simulink model "GFo_29bus"  (R2017b)
settings: Solver=ode1  StartTime=0.0  StopTime=4.5  FixedStep=Time_Step  RelTol=1e-3  EnableMultiTasking=on
PreLoadFcn:
  | Init_29bus;
InitFcn:
  | Init_29bus;
undefined symbols (not defined in the file): C_line, D1, D11, Delta, DX_DR, fb, fn, I_thresh_pu, Kp_Rvi_pu, Time_Step, VSC01_Cf, VSC01_Cf_pu, VSC01_Delta_P_Time_Step, VSC01_Delta_P_Value, VSC01_id0, VSC01_Lf, VSC01_Lf_pu, VSC01_Lt_pu, VSC01_mp1, VSC01_mp2, VSC01_mp3, VSC01_Pn, VSC01_R, VSC01_Rf, VSC01_Rf_pu, VSC01_Rt_pu, VSC01_Rv, VSC01_Sn, VSC01_T1, VSC01_T2, VSC01_Tr_PLL, VSC01_Udc_n, VSC01_Udcb, VSC01_Un1, VSC01_Un2, VSC01_W_LF, VSC01_wc1, VSC01_wc2, VSC01_wc3
libraries: powerlib x183, sps_avr x6, simulink x4, powerlib_meascontrol x2
(part 1 of 7)
Description:
  | Copyright 2008-2017 The MathWorks, Inc.
settings Model: Creator=MathWorks  LastModifiedBy=Frederic_Colas
settings DataIOCC: SaveFormat=StructureWithTime  SignalLoggingSaveFormat=ModelDataLogs  SaveOutput=off  SignalLogging=off  DSMLogging=off  SaveTime=off
settings OptimizationCC: ExpressionDepthLimit=2147483647  LifeSpan=inf
settings DebuggingCC: UnderspecifiedInitializationDetection=Classic  MergeDetectMultiDrivingBlocksExec=none  SolverPrmCheckMsg=warning  FcnCallInpInsideContextMsg=warning  UnconnectedInputMsg=none  UnconnectedOutputMsg=none  UnconnectedLineMsg=none  StateNameClashWarn=warning  SFUnexpectedBacktrackingDiag=warning  SFNoUnconditionalDefaultTransitionDiag=warning  SFExecutionAtInitializationDiag=none
settings HardwareCC: ProdBitPerPointer=32  ProdBitPerSizeT=32  ProdBitPerPtrDiffT=32  ProdLargestAtomicFloat=None  ProdIntDivRoundTo=Undefined  ProdEndianess=Unspecified  ProdWordSize=32  ProdHWDeviceType=32-bit Generic
settings ModelReferenceCC: PropagateSignalLabelsOutOfModel=off
settings CodeAppCC: StateflowObjectComments=on
settings GRTTargetCC: TargetLangStandard=C89/C90 (ANSI)  GeneratePreprocessorConditionals=Disable all  CombineOutputUpdateFcns=off  GRTInterface=on
settings ConfigComp: CovMetricSettings=dw  CovHtmlReporting=on  CovSaveCumulativeToWorkspaceVar=on  CovSaveSingleToWorkspaceVar=on  CovExternalEMLEnable=off  CovSFcnEnable=off
settings SimscapeCC: SimscapeNormalizeSystem=off

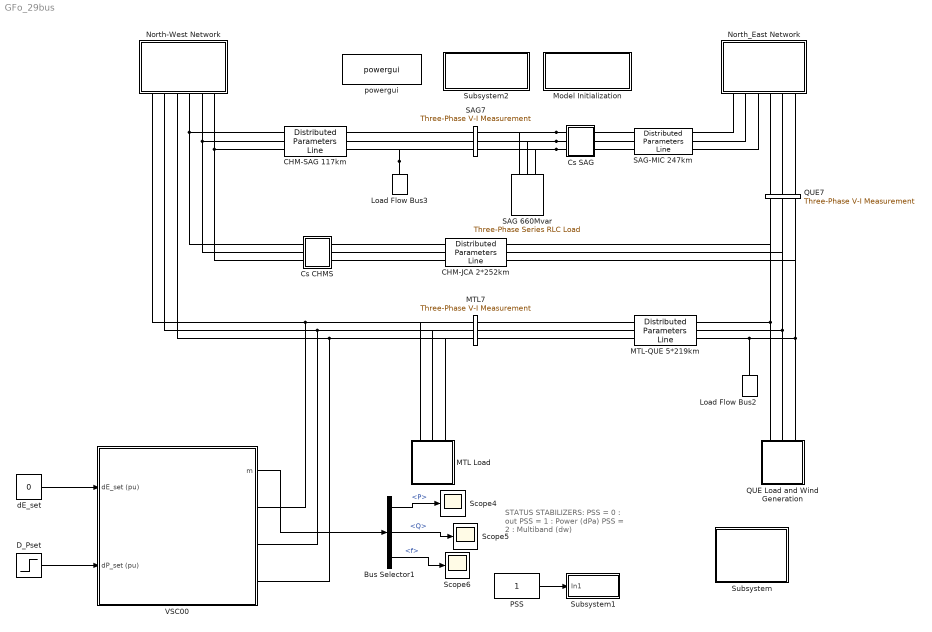
== system GFo_29bus ==
  note: STATUS STABILIZERS:
      | PSS = 0 :  out
      | PSS = 1 :  Power (dPa)
      | PSS = 2 :  Multiband (dw)
  Bus Selector1 : BusSelector  OutputSignals=control.P,control.Q,control.f
  CHM-JCA 2*252km : powerlib/Elements/Distributed Parameters Line  Phases=3  Frequency=60  Resistance="[0.01273  0.3864]/2"  Inductance="[0.9337e-3  4.1264e-3]/2"  Capacitance=[12.74e-9 7.751e-9]*2  Length=252  x1=[-0.00144 -3.02391793740978e-08 0 0;-0.0014 -3.09921305238755e-08 0 0;-0.00136 -3.17380343304367e-08 0 0;-0.00132 -3.24767211816884e-08 0 0;-0.00128 -3.32080231066107e-08 0 0;-0.00124 -3.39317738134523e-08 0 0;-0.0012 -3.46478087275439e-08 0 0;-0.00116 -3.53559650287208e-08 0 0;-0.00112 -3.60560816883471e-08 0 0;-0.00108 -3.67479995059318e-08 0 0;-0.00104 -3.74315611453301e-08 0 0;-0.001 -3.810661117052e-08 0 0;-0.00096 -3.87729960809472e-08 0 0;-0.00092 -3.94305643464296e-08 0 0;-0.00088 -4.00791664416144e-08 265077.167906972 -634102.982105748;-0.00084 -4.07186548799783e-08 274608.708093749 -630033.76126445;-0.0008 -4.13488842473653e-08 284077.80462843 -625821.276179022;-0.00076 -4.1969711235052e-08 293482.30432012 -621466.484732242;-0.00072 -4.25809946723352e-08 302820.068666693 -616970.377166134;-0.00068 -4.31825955586328e-08 312088.974341059 -612333.975856784;-0.00064 -4.37743770950913e-08 321286.913674001 -607558.335081867;-0.0006 -4.43562047156924e-08 330411.795133434 -602644.540780912;-0.00056 -4.49279461178528e-08 339461.543800003 -597593.710308369;-0.00052 -4.54894712925081e-08 348434.101838904 -592406.992179531;-0.00048 -4.6040652553676e-08 357327.428967815 -587085.565809372;-0.00044 -4.65813645674909e-08 366139.502920839 -581630.641244357;-0.0004 -4.71114843807037e-08 374868.319908351 -576043.458887293;-0.00036 -4.76308914486404e-08 383511.895072643 -570325.289215265;-0.00032 -4.81394676626131e-08 392068.262939261 -564477.432490745;-0.00028 -4.86370973767763e-08 400535.477863939 -558501.218465923;-0.00024 -4.91236674344246e-08 408911.614475022 -552398.006080331;-0.0002 -4.95990671937227e-08 417194.768111276 -546169.183151834;-0.00016 -5.00631885528651e-08 425383.055254997 -539816.166061051;-0.00012 -5.05159259746572e-08 433474.6139603 -533340.399429281;-8e-05 -5.09571765105133e-08 441467.604276514 -526743.355790014;-4e-05 -5.1386839823867e-08 449360.208666571 -520026.53525408]  x2=[-0.00144 -2.32746545563594e-08 0 0;-0.0014 -2.37082501505167e-08 0 0;-0.00136 -2.41364546930411e-08 0 0;-0.00132 -2.45591708139122e-08 0 0;-0.00128 -2.49763023911295e-08 0 0;-0.00124 -2.53877545725695e-08 0 0;-0.0012 -2.57934337975543e-08 0 0;-0.00116 -2.61932478181267e-08 0 0;-0.00112 -2.65871057200262e-08 0 0;-0.00108 -2.69749179433624e-08 0 0;-0.00104 -2.73565963029801e-08 0 0;-0.001 -2.77320540085117e-08 0 0;-0.00096 -2.81012056841128e-08 0 0;-0.00092 -2.84639673878759e-08 0 0;-0.00088 -2.88202566309177e-08 37345.2323788199 -657445.860812689;-0.00084 -2.9169992396137e-08 47254.6604347232 -656807.985703751;-0.0008 -2.95130951566367e-08 57153.3431883505 -656020.758122934;-0.00076 -2.98494868938078e-08 67039.0297646062 -655084.357079001;-0.00072 -3.01790911150703e-08 76909.4722436134 -653998.995501477;-0.00068 -3.05018328712667e-08 86762.4261718714 -652764.920192222;-0.00064 -3.08176387737047e-08 96595.6510726253 -651382.41176932;-0.0006 -3.11264370108456e-08 106406.910955331 -649851.784603265;-0.00056 -3.14281573646332e-08 116193.974824099 -648173.386745474;-0.00052 -3.17227312264609e-08 125954.617185006 -646347.599849146;-0.00048 -3.2010091612773e-08 135686.618552152 -644374.839082477;-0.00044 -3.22901731802955e-08 145387.765952351 -642255.553034253;-0.0004 -3.25629122408955e-08 155055.853428343 -639990.223611844;-0.00036 -3.28282467760625e-08 164688.68254041 -637579.365931627;-0.00032 -3.30861164510113e-08 174284.062866282 -635023.528201848;-0.00028 -3.33364626284017e-08 183839.81249922 -632323.291597964;-0.00024 -3.35792283816718e-08 193353.758544162 -629479.270130496;-0.0002 -3.38143585079829e-08 202823.737611824 -626492.110505397;-0.00016 -3.40417995407718e-08 212247.59631063 -623362.491977008;-0.00012 -3.42614997619092e-08 221623.19173638 -620091.126193592;-8e-05 -3.44734092134592e-08 230948.391959526 -616678.757035518;-4e-05 -3.46774797090402e-08 240221.076509955 -613126.160446105]  x3=[-0.00144 -1.32107929850916e-10 0 0;-0.0014 -1.33450786607546e-10 0 0;-0.00136 -1.34763297806132e-10 0 0;-0.00132 -1.36045164992946e-10 0 0;-0.00128 -1.37296096682445e-10 0 0;-0.00124 -1.38515808423548e-10 0 0;-0.0012 -1.39704022864326e-10 0 0;-0.00116 -1.4086046981506e-10 0 0;-0.00112 -1.41984886309688e-10 0 0;-0.00108 -1.43077016665594e-10 0 0;-0.00104 -1.44136612541754e-10 0 0;-0.001 -1.45163432995204e-10 0 0;-0.00096 -1.46157244535826e-10 0 0;-0.00092 -1.47117821179447e-10 0 0;-0.00088 -1.48044944499222e-10 455.51432786146 206.852095953411;-0.00084 -1.48938403675303e-10 452.343644908568 213.697505315651;-0.0008 -1.49797995542779e-10 449.07010291167 220.494321708032;-0.00076 -1.50623524637871e-10 445.694446245985 227.240999593118;-0.00072 -1.51414803242382e-10 442.217442506729 233.936004834539;-0.00068 -1.52171651426382e-10 438.639882334567 240.57781504584;-0.00064 -1.5289389708912e-10 434.962579235833 247.164919936653;-0.0006 -1.5358137599816e-10 431.186369397537 253.695821656133;-0.00056 -1.54233931826728e-10 427.312111497233 260.169035133548;-0.00052 -1.54851416189255e-10 423.340686507758 266.583088415975;-0.00048 -1.55433688675123e-10 419.272997496905 272.936523003011;-0.00044 -1.55980616880589e-10 415.109969422078 279.227894178421;-0.0004 -1.56492076438896e-10 410.85254891996 285.455771338653;-0.00036 -1.5696795104855e-10 406.501704091259 291.618738318149;-0.00032 -1.57408132499771e-10 402.05842428057 297.715393711364;-0.00028 -1.5781252069909e-10 397.523719851403 303.744351191437;-0.00024 -1.5818102369212e-10 392.89862195644 309.704239825429;-0.0002 -1.58513557684458e-10 388.184182303058 315.593704386061;-0.00016 -1.58810047060741e-10 383.381472914178 321.411405659879;-0.00012 -1.59070424401841e-10 378.491585884498 327.156020751784;-8e-05 -1.59294630500198e-10 373.515633132161 332.826243385843;-4e-05 -1.59482614373277e-10 368.454746145911 338.420784202328]  x4=[-0.00144 5.44626892198022e-11 0 0;-0.0014 5.22863667553336e-11 0 0;-0.00136 5.00981548219633e-11 0 0;-0.00132 4.78985510002146e-11 0 0;-0.00128 4.56880554610279e-11 0 0;-0.00124 4.34671708520264e-11 0 0;-0.0012 4.12364021832181e-11 0 0;-0.00116 3.89962567121609e-11 0 0;-0.00112 3.67472438286167e-11 0 0;-0.00108 3.44898749387207e-11 0 0;-0.00104 3.22246633486916e-11 0 0;-0.001 2.99521241481107e-11 0 0;-0.00096 2.76727740927946e-11 0 0;-0.00092 2.53871314872896e-11 0 0;-0.00088 2.30957160670137e-11 190.753638286441 -10030.4733717918;-0.00084 2.07990488800732e-11 341.981891608961 -10026.4567433659;-0.0008 1.84976521687807e-11 493.132381198454 -10020.1601851409;-0.00076 1.6192049250902e-11 644.170736737055 -10011.5851289001;-0.00072 1.38827644006579e-11 795.062613405215 -10000.7335245372;-0.00068 1.15703227295089e-11 945.773699691414 -9987.60783961345;-0.00064 9.2552500667495e-12 1096.26972519431 -9972.21105879643;-0.0006 6.93807283993878e-12 1246.51646841552 -9954.54668318134;-0.00056 4.61931795519565e-12 1396.47976454132 -9934.61872949484;-0.00052 2.29951267738481e-12 1546.12551321138 -9912.43172918176;-0.00048 -2.08154897787282e-14 1695.41968627296 -9887.99072737463;-0.00044 -2.34113892367939e-12 1844.32833551856 -9861.3012817465;-0.0004 -4.66093000277792e-12 1992.81760040548 -9832.36946124714;-0.00036 -6.97966122658797e-12 2140.85371575538 -9801.20184472303;-0.00032 -9.29680533562514e-12 2288.40301943227 -9767.8055194214;-0.00028 -1.16118354313012e-11 2435.43195999687 -9732.18807937862;-0.00024 -1.39242250957364e-11 2581.90710433605 -9694.35762369341;-0.0002 -1.62334485114622e-11 2727.79514526512 -9654.32275468515;-0.00016 -1.85389805809879e-11 2873.06290910166 -9612.0925759378;-0.00012 -2.08402970462027e-11 3017.67736320891 -9567.67669022985;-8e-05 -2.31368746075884e-11 3161.60562350711 -9521.08519735066;-4e-05 -2.54281910432121e-11 3304.81496195104 -9472.32869180394]  x5=0.00142516474882927  V1=ones(3,3)  V2=ones(3,3)  I1=ones(3,3)  I2=ones(3,3)  nHarmo=1  Measurements=None
      settings: AttributesFormatString=\n  SourceProductName=Simscape Power Systems
  CHM-SAG 117km : powerlib/Elements/Distributed Parameters Line  Phases=3  Frequency=60  Resistance="[0.01273  0.3864]"  Inductance="[0.9337e-3  4.1264e-3]"  Capacitance=[12.74e-9 7.751e-9]  Length=117  x1=[-0.00068 -4.23803703751889e-08 0 0;-0.00064 -4.29595449086164e-08 0 0;-0.0006 -4.35289508119991e-08 0 0;-0.00056 -4.40884586073449e-08 0 0;-0.00052 -4.4637941067406e-08 0 0;-0.00048 -4.51772732446096e-08 0 0;-0.00044 -4.57063324994695e-08 290815.275178508 -619240.212617567;-0.0004 -4.62249985284737e-08 300119.775081889 -614784.578978232;-0.00036 -4.673315339144e-08 309356.030336538 -610189.148627313;-0.00032 -4.72306815383346e-08 318521.940697662 -605454.966526043;-0.00028 -4.77174698355474e-08 327615.421916287 -600583.109186607;-0.00024 -4.81934075916175e-08 336634.406213204 -595574.68442735;-0.0002 -4.86583865824036e-08 345576.842749159 -590430.831120871;-0.00016 -4.91123010756929e-08 354440.698091201 -585152.718935054;-0.00012 -4.9555047855244e-08 363223.956675063 -579741.548067093;-8e-05 -4.99865262442574e-08 371924.621263487 -574198.54897058;-4e-05 -5.04066381282682e-08 380540.713400378 -568524.982075709]  x2=[-0.00068 -2.9225958888399e-08 0 0;-0.00064 -2.96330480824069e-08 0 0;-0.0006 -3.00333989768254e-08 0 0;-0.00056 -3.04269205353136e-08 0 0;-0.00052 -3.08135232744627e-08 0 0;-0.00048 -3.11931192841436e-08 0 0;-0.00044 -3.15656222474974e-08 342715.137788314 -587516.495420752;-0.0004 -3.19309474605624e-08 351535.375086538 -582281.875650636;-0.00036 -3.22890118515356e-08 360275.676271978 -576914.850003381;-0.00032 -3.26397339996624e-08 368934.05387552 -571416.638894338;-0.00028 -3.29830341537507e-08 377508.539056762 -565788.492569297;-0.00024 -3.3318834250306e-08 385997.182051718 -560031.690820198;-0.0002 -3.36470579312822e-08 394398.052616172 -554147.542694114;-0.00016 -3.39676305614447e-08 402709.240464606 -548137.386195587;-0.00012 -3.42804792453419e-08 410928.855704575 -542002.587982374;-8e-05 -3.45855328438809e-08 419055.029266456 -535744.543054685;-4e-05 -3.48827219905042e-08 427085.913328459 -529364.67443797]  x3=[-0.00068 -9.13993390137404e-11 0 0;-0.00064 -9.10085517468096e-11 0 0;-0.0006 -9.0597069920036e-11 0 0;-0.00056 -9.01649871008385e-11 0 0;-0.00052 -8.97124015411239e-11 0 0;-0.00048 -8.92394161549457e-11 0 0;-0.00044 -8.87461384951018e-11 1711.45288043998 -3591.83174853406;-0.0004 -8.82326807286782e-11 1765.41999013625 -3565.61618486843;-0.00036 -8.76991596115431e-11 1818.9856585511 -3538.58983083092;-0.00032 -8.71456964617978e-11 1872.13770531345 -3510.75883198137;-0.00028 -8.65724171321895e-11 1924.86404410625 -3482.12951684893;-0.00024 -8.5979451981494e-11 1977.15268541473 -3452.70839549296;-0.0002 -8.53669358448732e-11 2028.99173925279 -3422.50215802275;-0.00016 -8.47350080032144e-11 2080.36941786663 -3391.51767307621;-0.00012 -8.40838121514592e-11 2131.27403841518 -3359.761986258;-8e-05 -8.34134963659287e-11 2181.69402562672 -3327.24231853748;-4e-05 -8.27242130706519e-11 2231.61791443097 -3293.96606460664]  x4=[-0.00068 9.30343370038175e-12 0 0;-0.00064 7.45357527579132e-12 0 0;-0.0006 5.60202197246008e-12 0 0;-0.00056 3.74919481764209e-12 0 0;-0.00052 1.89551512825424e-12 0 0;-0.00048 4.14044150724481e-14 0 0;-0.00044 -1.81271571311628e-12 280.288551649878 -1025.23386773629;-0.0004 -3.66642364538403e-12 295.716038711893 -1020.89088180168;-0.00036 -5.51929786453271e-12 311.076282496852 -1016.31575408433;-0.00032 -7.3709170429434e-12 326.365790217779 -1011.50952492885;-0.00028 -9.22086013838259e-12 341.581085172469 -1006.47328723028;-0.00024 -1.10687064897436e-11 356.71870753406 -1001.20818618565;-0.0002 -1.29140359127014e-11 371.775215137769 -995.71541903353;-0.00016 -1.47564287952585e-11 386.747184263609 -989.996234781809;-0.00012 -1.65954661931615e-11 401.631210414913 -984.051933923662;-8e-05 -1.84307299251655e-11 416.423909092489 -977.883868141844;-4e-05 -2.02618026681243e-11 431.121916564223 -971.493440001321]  x5=0.000661683633385019  V1=ones(3,3)  V2=ones(3,3)  I1=ones(3,3)  I2=ones(3,3)  nHarmo=1  Measurements=None
      settings: AttributesFormatString=\n  SourceProductName=Simscape Power Systems
  Cs CHMS : Subsystem  mask{Xc=33/2}
      mask prompts: Xc "Condensator Reactance at  60Hz  (ohm):"
      mask help: Series Compensation
      mask init:
      | Cs=1/Xc/(2*pi*60);
      mask Display: disp('Cs')
  Cs SAG : Subsystem  mask{Xc=22}
      mask prompts: Xc "Condensator Reactance at  60Hz  (ohm):"
      mask help: Series Compensation
      mask init:
      | Cs=1/Xc/(2*pi*60);
      mask Display: disp('Cs')
  D_Pset : Step  Time=VSC01_Delta_P_Time_Step  After=VSC01_Delta_P_Value  SampleTime=0
  Load Flow Bus2 : powerlib/Measurements/Load Flow Bus  LConnTagsString=a  Phases=single  Connectors=on one side  ID=QUE7  Vbase=735e3  Vref=1  Vangle=0  VLF=1.016  VLFb=1  VLFc=1  angleLF=-12.43  angleLFb=0  angleLFc=0
      settings: AttributesFormatString=%<ID>\n%<Vbase>V\n%<VLF>pu\n%<angleLF>deg.  SourceProductName=Simscape Power Systems
  Load Flow Bus3 : powerlib/Measurements/Load Flow Bus  LConnTagsString=a  Phases=single  Connectors=on one side  ID=SAG7  Vbase=735e3  Vref=1  Vangle=0  VLF=1.034  VLFb=1  VLFc=1  angleLF=2.226  angleLFb=0  angleLFc=0
      settings: AttributesFormatString=%<ID>\n%<Vbase>V\n%<VLF>pu\n%<angleLF>deg.  SourceProductName=Simscape Power Systems
  MTL Load : Subsystem
  MTL-QUE 5*219km : powerlib/Elements/Distributed Parameters Line  Phases=3  Frequency=60  Resistance="[0.01273  0.3864]/5"  Inductance="[0.9337e-3  4.1264e-3]/5"  Capacitance=[12.74e-9 7.751e-9]*5  Length=219  x1=[-0.00124 -1.29467243971328e-07 -185501.595169669 -635267.89625739;-0.0012 -1.3225224728807e-07 -175901.255117953 -637992.862327818;-0.00116 -1.35007177584273e-07 -166260.91663773 -640572.754323168;-0.00112 -1.37731408412545e-07 -156582.771858837 -643006.985598249;-0.00108 -1.4042432030629e-07 -146869.021507936 -645295.002629861;-0.00104 -1.43085300920565e-07 -137121.874408088 -647436.285142663;-0.001 -1.45713745171325e-07 -127343.546976489 -649430.346227476;-0.00096 -1.48309055373016e-07 -117536.262720471 -651276.732452005;-0.00092 -1.50870641374477e-07 -107702.2517319 -652975.023963946;-0.00088 -1.53397920693143e-07 -97843.7501800699 -654524.834586454;-0.00084 -1.55890318647491e-07 -87962.9998032174 -655925.81190596;-0.0008 -1.58347268487719e-07 -78062.2473987702 -657177.637352301;-0.00076 -1.60768211524621e-07 -68143.7443124447 -658280.026271167;-0.00072 -1.63152597256629e-07 -58209.7459263092 -659232.727988824;-0.00068 -1.65499883494989e-07 -48262.5111459295 -660035.525869117;-0.00064 -1.67809536487052e-07 -38304.3018867134 -660688.237362731;-0.0006 -1.70081031037646e-07 -28337.3825595705 -661190.714048703;-0.00056 -1.72313850628499e-07 -18364.0195560047 -661542.841668165;-0.00052 -1.74507487535689e-07 -8386.48073275649 -661744.540150334;-0.00048 -1.76661442945103e-07 1592.96510388849 -661795.763630715;-0.00044 -1.78775227065854e-07 11572.048714006 -661696.50046153;-0.0004 -1.80848359241663e-07 21548.500940039 -661446.773214367;-0.00036 -1.82880368060149e-07 31520.0532227846 -661046.63867505;-0.00032 -1.84870791460032e-07 41484.4381172447 -660496.187830721;-0.00028 -1.86819176836195e-07 51439.3898082235 -659795.545849157;-0.00024 -1.88725081142605e-07 61382.6446255543 -658944.8720503;-0.0002 -1.90588070993059e-07 71311.9415588386 -657944.359870038;-0.00016 -1.92407722759731e-07 81225.0227715805 -656794.236816212;-0.00012 -1.94183622669501e-07 91119.6341145989 -655494.764416886;-8e-05 -1.95915366898044e-07 100993.525638602 -654046.238160878;-4e-05 -1.97602561661656e-07 110844.452105806 -652448.987430567]  x2=[-0.00124 -2.53877545725695e-08 -51950.9609807774 -656453.169013363;-0.0012 -2.57934337975543e-08 -42046.3485068077 -657161.91059321;-0.00116 -2.61932478181267e-08 -32132.1750557799 -657721.219221712;-0.00112 -2.65871057200262e-08 -22210.6950252404 -658130.967716908;-0.00108 -2.69749179433624e-08 -12284.1644741892 -658391.062905526;-0.00104 -2.73565963029801e-08 -2354.84061007062 -658501.445644162;-0.001 -2.77320540085117e-08 7575.01872449539 -658462.090832732;-0.00096 -2.81012056841128e-08 17503.1555651277 -658273.007420183;-0.00092 -2.84639673878759e-08 27427.3123391252 -657934.238402451;-0.00088 -2.88202566309177e-08 37345.2323788199 -657445.860812689;-0.00084 -2.9169992396137e-08 47254.6604347232 -656807.985703751;-0.0008 -2.95130951566367e-08 57153.3431883505 -656020.758122934;-0.00076 -2.98494868938078e-08 67039.0297646062 -655084.357079001;-0.00072 -3.01790911150703e-08 76909.4722436134 -653998.995501477;-0.00068 -3.05018328712667e-08 86762.4261718714 -652764.920192222;-0.00064 -3.08176387737047e-08 96595.6510726253 -651382.41176932;-0.0006 -3.11264370108456e-08 106406.910955331 -649851.784603265;-0.00056 -3.14281573646332e-08 116193.974824099 -648173.386745474;-0.00052 -3.17227312264609e-08 125954.617185006 -646347.599849146;-0.00048 -3.2010091612773e-08 135686.618552152 -644374.839082477;-0.00044 -3.22901731802955e-08 145387.765952351 -642255.553034253;-0.0004 -3.25629122408955e-08 155055.853428343 -639990.223611844;-0.00036 -3.28282467760625e-08 164688.68254041 -637579.365931627;-0.00032 -3.30861164510113e-08 174284.062866282 -635023.528201848;-0.00028 -3.33364626284017e-08 183839.81249922 -632323.291597964;-0.00024 -3.35792283816718e-08 193353.758544162 -629479.270130496;-0.0002 -3.38143585079829e-08 202823.737611824 -626492.110505397;-0.00016 -3.40417995407718e-08 212247.59631063 -623362.491977008;-0.00012 -3.42614997619092e-08 221623.19173638 -620091.126193592;-8e-05 -3.44734092134592e-08 230948.391959526 -616678.757035518;-4e-05 -3.46774797090402e-08 240221.076509955 -613126.160446105]  x3=[-0.00124 -2.34539964048353e-09 -6146.56877360705 -19926.8976541734;-0.0012 -2.33672238628343e-09 -5845.39055122427 -20017.3164990862;-0.00116 -2.32751378156371e-09 -5542.88313743863 -20103.1835788491;-0.00112 -2.31777592028169e-09 -5239.11531982733 -20184.4793680287;-0.00108 -2.30751101674305e-09 -4934.15617257251 -20261.1853806635;-0.00104 -2.29672140509833e-09 -4628.07504075439 -20333.2841744677;-0.001 -2.28540953881217e-09 -4320.94152458283 -20400.7593547975;-0.00096 -2.27357799010542e-09 -4012.82546357079 -20463.5955783786;-0.00092 -2.26122944937022e-09 -3703.79692065347 -20521.7785567958;-0.00088 -2.24836672455824e-09 -3393.92616625657 -20575.2950597414;-0.00084 -2.23499274054219e-09 -3083.28366231744 -20624.1329180242;-0.0008 -2.2211105384507e-09 -2771.9400462626 -20668.2810263364;-0.00076 -2.2067232749768e-09 -2459.96611494544 -20707.7293457789;-0.00072 -2.19183422166015e-09 -2147.43280854758 -20742.468906144;-0.00068 -2.17644676414306e-09 -1834.41119444774 -20772.4918079552;-0.00064 -2.16056440140069e-09 -1520.97245106156 -20797.7912242637;-0.0006 -2.14419074494535e-09 -1207.18785165632 -20818.3614022003;-0.00056 -2.12732951800532e-09 -893.128748143954 -20834.197664284;-0.00052 -2.10998455467821e-09 -578.866554856277 -20845.2964094852;-0.00048 -2.09215979905909e-09 -264.472732305958 -20851.6551140451;-0.00044 -2.07385930434369e-09 49.9812290629714 -20853.2723320491;-0.0004 -2.05508723190668e-09 364.423825131431 -20850.1476957558;-0.00036 -2.03584785035545e-09 678.783554364714 -20842.2819156804;-0.00032 -2.01614553455946e-09 992.988934071314 -20829.6767804337;-0.00028 -1.9959847646554e-09 1306.96851665748 -20812.3351563145;-0.00024 -1.9753701250285e-09 1620.65090587377 -20790.2609866587;-0.0002 -1.95430630327004e-09 1933.96477304997 -20763.4592909421;-0.00016 -1.93279808911143e-09 2246.83887331457 -20731.9361636392;-0.00012 -1.9108503733351e-09 2559.2020617953 -20695.6987728373;-8e-05 -1.88846814666235e-09 2870.98330979679 -20654.7553586066;-4e-05 -1.8656564986185e-09 3182.11172095194 -20609.1152311263]  x4=[-0.00124 1.70103533998812e-09 -1607.3065331276 -3120.16619531001;-0.0012 1.66868321752917e-09 -1560.07481785239 -3144.04837089683;-0.00116 1.63595165089666e-09 -1512.4883550171 -3167.21561699723;-0.00112 1.60284808296658e-09 -1464.55796537303 -3189.66266557923;-0.00108 1.56938004120481e-09 -1416.29454787745 -3211.38441237756;-0.00104 1.53555513595542e-09 -1367.70907721528 -3232.37591805431;-0.001 1.50138105871019e-09 -1318.81260130357 -3252.63240932212;-0.00096 1.46686558035956e-09 -1269.61623877928 -3272.14928002956;-0.00092 1.43201654942567e-09 -1220.131176471 -3290.92209220853;-0.00088 1.39684189027762e-09 -1170.36866685515 -3308.94657708343;-0.00084 1.36134960132957e-09 -1120.34002549729 -3326.21863604185;-0.0008 1.32554775322197e-09 -1070.05662847902 -3342.73434156652;-0.00076 1.28944448698631e-09 -1019.52990981122 -3358.48993812843;-0.00072 1.25304801219401e-09 -968.771358833984 -3373.4818430408;-0.00068 1.21636660508957e-09 -917.792517604073 -3387.70664727372;-0.00064 1.17940860670862e-09 -866.604978270365 -3401.16111622939;-0.0006 1.1421824209813e-09 -815.220380437881 -3413.8421904776;-0.00056 1.10469651282121e-09 -763.650408521046 -3425.74698645141;-0.00052 1.06695940620059e-09 -711.906789086755 -3436.87279710289;-0.00048 1.02897968221208e-09 -660.001288187848 -3447.21709251864;-0.00044 9.90765977117372e-10 -607.945708687615 -3456.77752049508;-0.0004 9.5232698038347e-10 -555.751887575928 -3465.55190707334;-0.00036 9.13671432706747e-10 -503.431693277606 -3473.53825703358;-0.00032 8.74808124025393e-10 -450.997022953643 -3480.73475434868;-0.00028 8.3574589152066e-10 -398.459799795892 -3487.13976259723;-0.00024 7.9649361760736e-10 -345.831970315839 -3492.75182533557;-0.0002 7.57060227914085e-10 -293.125501628065 -3497.56966642904;-0.00016 7.17454689253592e-10 -240.352378729026 -3501.59219034213;-0.00012 6.77686007583828e-10 -187.524601771776 -3504.81848238757;-8e-05 6.37763225960055e-10 -134.654183337225 -3507.24780893438;-4e-05 5.97695422478535e-10 -81.7531457025922 -3508.87961757467]  x5=0.00123853603172068  V1=ones(3,3)  V2=ones(3,3)  I1=ones(3,3)  I2=ones(3,3)  nHarmo=1  Measurements=None
      settings: AttributesFormatString=\n  SourceProductName=Simscape Power Systems
  MTL7 : powerlib/Measurements/Three-Phase V-I Measurement  VoltageMeasurement=phase-to-ground  SetLabelV=on  LabelV=Vabc_MTL7  Vpu=on  VpuLL=off  CurrentMeasurement=no  SetLabelI=off  LabelI=A1  Ipu=off  Pbase=100e6  Vbase=735e3  OutputType=Magnitude  PhasorSimulation=off  PSBequivalent=0
  Model Initialization : Subsystem  mask(Model Functions){InitFcnX=Init_29bus;, prel=on, posl=off, inif=on, strf=off}
      mask prompts: InitFcnX "Initialisation"; prel "Preload Function"; posl "PostLoad Function"; inif "InitFcn"; strf "StartFcn"
      mask init:
      | currentBlock = gcb;
      | root = bdroot(currentBlock);
      | 
      | if ~strcmp(get_param(root,'BlockDiagramType'),'library')
      |     if prel==1
      |         set_param(root, 'PreLoadFcn', InitFcnX);
      |     else
      |         set_param(root, 'PreLoadFcn', '');
      |     end
      |     if inif==1
      |         set_param(root, 'InitFcn', InitFcnX);
      |     else
      |         set_param(root, 'InitFcn', '');
      |     end
      |     if strf==1
      |         set_param(root, 'StartFcn', InitFcnX);
      |     else
      |         set_param(root, 'StartFcn', '');
      |     end
      |     if posl==1
      |         set_param(root, 'PostLoadFcn', InitFcnX);
      |     else
      |         set_param(root, 'PostLoadFcn', '');
      |     end
      | end
      | 
      | pos = get_param(currentBlock, 'Position');
      | width = pos(3) - pos(1); height = pos(4) - pos(2);
      | txt = [ upper(root) '\n' '- InitFcn. . . . . '  get_param(root, 'InitFcn') ];
      settings: CopyFcn=set_param(gcb,'LinkStatus','none')
      mask Display:
      | %text(5, height*0.5, txt, 'horizontalAlignment', 'left', 'verticalAlignment', 'middle') ;
      | color('blue'),disp('Initialization Function\nParameters')
  North-West Network : Subsystem
  North_East Network : Subsystem
  PSS : Constant
  QUE Load and Wind Generation : Subsystem
  QUE7 : powerlib/Measurements/Three-Phase V-I Measurement  VoltageMeasurement=no  SetLabelV=on  LabelV=Vabc_QUE7  Vpu=on  VpuLL=off  CurrentMeasurement=no  SetLabelI=off  LabelI=A1  Ipu=off  Pbase=100e6  Vbase=735e3  OutputType=Magnitude  PhasorSimulation=off  PSBequivalent=0
  SAG 660Mvar : powerlib/Elements/Three-Phase Series RLC Load  LConnTagsString=A|B|C  Configuration=Y (grounded)  NominalVoltage=735e3  Vabc=[1e3 1e3 1e3]  Vabcp=[1e3 1e3 1e3]  NominalFrequency=60  UnbalancedPower=off  ActivePower=2200000  InductivePower=660e6  CapacitivePower=0  Pabc=[10e3 9e3 11e3]  QLabc=[100 90 110]  QCabc=[100 90 110]  Pabcp=[10e3 9e3 11e3]  QLabcp=[100 90 110]  QCabcp=[100 90 110]  Measurements=None  LoadType=constant Z
  SAG-MIC 247km : powerlib/Elements/Distributed Parameters Line  Phases=3  Frequency=60  Resistance="[0.01273  0.3864]/1"  Inductance="[0.9337e-3  4.1264e-3]/1"  Capacitance=[12.74e-9 7.751e-9]*1  Length=247  x1=[-0.0014 -2.18287772271905e-08 78316.7403979905 -664135.918195675;-0.00136 -2.23509066790489e-08 88322.3876580945 -662879.466032313;-0.00132 -2.28679537274745e-08 98307.9511689049 -661472.280794804;-0.00128 -2.33798008004273e-08 108271.160299391 -659914.682464936;-0.00124 -2.3886331508297e-08 118209.749501716 -658207.025227138;-0.0012 -2.43874306703686e-08 128121.458826402 -656349.697387939;-0.00116 -2.4882984341014e-08 138004.034436223 -654343.121287672;-0.00112 -2.53728798356019e-08 147855.229118709 -652187.753204439;-0.00108 -2.58570057561217e-08 157672.802797143 -649884.083250356;-0.00104 -2.63352520165138e-08 167454.523039933 -647432.635260102;-0.001 -2.68075098677029e-08 177198.16556825 -644833.966671812;-0.00096 -2.72736719223262e-08 186901.514761809 -642088.668400312;-0.00092 -2.77336321791525e-08 196562.364162681 -639197.364702755;-0.00088 -2.8187286047186e-08 206178.516977024 -636160.713036668;-0.00084 -2.86345303694491e-08 215747.786574614 -632979.403910452;-0.0008 -2.90752634464398e-08 225267.996986067 -629654.160726369;-0.00076 -2.95093850592572e-08 234736.983397634 -626185.739616043;-0.00072 -2.99367964923903e-08 244152.592643461 -622574.929268524;-0.00068 -3.03574005561649e-08 253512.683695204 -618822.550750947;-0.00064 -3.07711016088441e-08 262815.128148875 -614929.457321828;-0.0006 -3.11778055783762e-08 272057.810708826 -610896.53423704;-0.00056 -3.15774199837857e-08 281238.629668748 -606724.698548513;-0.00052 -3.19698539562029e-08 290355.497389582 -602414.898895707;-0.00048 -3.23550182595268e-08 299406.340774229 -597968.115289898;-0.00044 -3.27328253107162e-08 308389.101738955 -593385.358891328;-0.0004 -3.31031891997059e-08 317301.737681379 -588667.671779285;-0.00036 -3.34660257089412e-08 326142.221944948 -583816.126715132;-0.00032 -3.38212523325291e-08 334908.544279777 -578831.82689838;-0.00028 -3.41687882949987e-08 343598.711299766 -573715.905715825;-0.00024 -3.4508554569669e-08 352210.746935874 -568469.526483825;-0.0002 -3.48404738966193e-08 360742.692885465 -563093.882183775;-0.00016 -3.51644708002569e-08 369192.609057607 -557590.195190832;-0.00012 -3.54804716064801e-08 377558.57401423 -551959.716995955;-8e-05 -3.57884044594304e-08 385838.685407048 -546203.727921331;-4e-05 -3.60881993378328e-08 394031.060410137 -540323.536829238]  x2=[-0.0014 -6.63956079804801e-09 207386.670092934 -660622.377543572;-0.00136 -6.78555895187547e-09 217324.673149015 -657420.085739957;-0.00132 -6.93001412811345e-09 227213.258448551 -654068.302278195;-0.00128 -7.07289347890059e-09 237050.177412518 -650567.789324939;-0.00124 -7.21416451470466e-09 246833.193210376 -646919.342866648;-0.0012 -7.35379511171039e-09 256560.081268697 -643123.792528584;-0.00116 -7.49175351912415e-09 266228.629777017 -639182.001386163;-0.00112 -7.62800836639379e-09 275836.640190783 -635094.865768697;-0.00108 -7.76252867034205e-09 285381.927731285 -630863.31505558;-0.00104 -7.89528384221188e-09 294862.321882449 -626488.311464953;-0.001 -8.02624369462201e-09 304275.666884401 -621970.849834905;-0.00096 -8.15537844843136e-09 313619.822223665 -617311.957397252;-0.00092 -8.28265873951053e-09 322892.663119898 -612512.693543958;-0.00088 -8.40805562541895e-09 332092.081009045 -607574.149586237;-0.00084 -8.53154059198612e-09 341215.984022811 -602497.448506396;-0.0008 -8.65308555979555e-09 350262.297464331 -597283.744702482;-0.00076 -8.77266289056971e-09 359228.964279942 -591934.223725778;-0.00072 -8.89024539345479e-09 368113.945526933 -586450.102011222;-0.00068 -9.0058063312036e-09 376915.220837192 -580832.626600799;-0.00064 -9.11931942625546e-09 385630.78887661 -575083.074859974;-0.0006 -9.23075886671145e-09 394258.667800176 -569202.754187231;-0.00056 -9.34009931220383e-09 402796.895702627 -563193.001716782;-0.00052 -9.44731589965819e-09 411243.531064567 -557055.184014512;-0.00048 -9.55238424894716e-09 419596.653193956 -550790.696767236;-0.00044 -9.65528046843417e-09 427854.362662856 -544400.964465332;-0.0004 -9.75598116040625e-09 436014.781739346 -537887.440078822;-0.00036 -9.85446342639445e-09 444076.054814499 -531251.604726983;-0.00032 -9.95070487238077e-09 452036.348824337 -524494.967341547;-0.00028 -1.00446836138903e-08 459893.853666647 -517619.064323589;-0.00024 -1.01363782809677e-08 467646.782612589 -510625.459194162;-0.0002 -1.02257680230365e-08 475293.372712979 -503515.742238759;-0.00016 -1.031283251364e-08 482831.88519917 -496291.530145707;-0.00012 -1.03975519550641e-08 490260.605878431 -488954.465638535;-8e-05 -1.04799070828382e-08 497577.845523743 -481506.217102441;-4e-05 -1.05598791701166e-08 504781.940257911 -473948.478204911]  x3=[-0.0014 -6.73353084562707e-11 -14.414084581955 -3976.60584706905;-0.00136 -6.73420095932703e-11 45.5512644890894 -3976.37095443902;-0.00132 -6.73333977380212e-11 105.506255595407 -3975.23186934471;-0.00128 -6.7309474848785e-11 165.437255489049 -3973.18885080424;-0.00124 -6.72702463654203e-11 225.330636377463 -3970.24236338243;-0.0012 -6.72157212081461e-11 285.172779022333 -3966.3930770851;-0.00116 -6.71459117755127e-11 344.950075836479 -3961.64186720675;-0.00112 -6.70608339415834e-11 404.648933978103 -3955.98981413155;-0.00108 -6.69605070523237e-11 464.255778441683 -3949.43820308761;-0.00104 -6.68449539212031e-11 523.757055144818 -3941.9885238548;-0.001 -6.67142008240072e-11 583.1392340103 -3933.64247042593;-0.00096 -6.65682774928627e-11 642.388812042748 -3924.40194062156;-0.00092 -6.64072171094766e-11 701.492316399062 -3914.2690356585;-0.00088 -6.62310562975913e-11 760.43630745204 -3903.24605967196;-0.00084 -6.60398351146563e-11 819.207381846426 -3891.3355191916;-0.0008 -6.58335970427195e-11 877.792175546723 -3878.54012257162;-0.00076 -6.56123889785399e-11 936.177366876059 -3864.86277937488;-0.00072 -6.53762612229237e-11 994.349679545417 -3850.30659971127;-0.00068 -6.51252674692863e-11 1052.29588567255 -3834.87489353051;-0.00064 -6.48594647914428e-11 1110.0028087899 -3818.57116986951;-0.0006 -6.45789136306299e-11 1167.45732684078 -3801.39913605445;-0.00056 -6.42836777817622e-11 1224.64637516327 -3783.36269685771;-0.00052 -6.39738243789258e-11 1281.55694946094 -3764.46595361004;-0.00048 -6.36494238801124e-11 1338.17610875998 -3744.71320326789;-0.00044 -6.33105500511979e-11 1394.49097835183 -3724.10893743635;-0.0004 -6.29572799491687e-11 1450.48875272078 -3702.65784134778;-0.00036 -6.25896939045995e-11 1506.15669845585 -3680.36479279645;-0.00032 -6.22078755033869e-11 1561.48215714622 -3657.23486102935;-0.00028 -6.18119115677428e-11 1616.45254825971 -3633.27330559351;-0.00024 -6.14018921364513e-11 1671.05537200342 -3608.48557513999;-0.0002 -6.09779104443954e-11 1725.2782121661 -3582.87730618493;-0.00016 -6.05400629013555e-11 1779.10873894151 -3556.45432182787;-0.00012 -6.00884490700872e-11 1832.53471173205 -3529.22263042758;-8e-05 -5.9623171643681e-11 1885.54398193226 -3501.18842423585;-4e-05 -5.91443364222114e-11 1938.12449569121 -3472.35807798941]  x4=[-0.0014 4.77935028245795e-11 272.51466534708 -1044.02774481271;-0.00136 4.67968108426649e-11 288.226506380926 -1039.7999576739;-0.00132 4.57894776695232e-11 303.872807192781 -1035.33572899157;-0.00128 4.47717323640311e-11 319.450009948768 -1030.63607389283;-0.00124 4.37438063526944e-11 334.954572527312 -1025.7020610387;-0.0012 4.27059333770236e-11 350.382969324588 -1020.53481238117;-0.00116 4.16583494403831e-11 365.731692056214 -1015.13550290803;-0.00112 4.06012927543262e-11 380.997250555002 -1009.50536037568;-0.00108 3.95350036844276e-11 396.176173564594 -1003.64566502998;-0.00104 3.84597246956266e-11 411.265009528796 -997.55774931513;-0.001 3.73757002970922e-11 426.260327376429 -991.242997570655;-0.00096 3.62831769866247e-11 441.158717301529 -984.702845716648;-0.00092 3.51824031946031e-11 455.956791538705 -977.93878092724;-0.00088 3.40736292274953e-11 470.65118513349 -970.952341292435;-0.00084 3.29571072109395e-11 485.238556707498 -963.745115468356;-0.0008 3.1833091032414e-11 499.71558921823 -956.318742316003;-0.00076 3.07018362835046e-11 514.078990713337 -948.674910528589;-0.00072 2.95636002017857e-11 528.325495079185 -940.815358247546;-0.00068 2.84186416123266e-11 542.451862783537 -932.741872667282;-0.00064 2.72672208688367e-11 556.454881612197 -924.456289628798;-0.0006 2.61095997944637e-11 570.331367399441 -915.960493202223;-0.00056 2.49460416222571e-11 584.078164752067 -907.256415258401;-0.00052 2.37768109353111e-11 597.692147766903 -898.346035029596;-0.00048 2.26021736066009e-11 611.170220741616 -889.231378659431;-0.00044 2.14223967385254e-11 624.509318878639 -879.914518742164;-0.0004 2.02377486021704e-11 637.706408982088 -870.397573851394;-0.00036 1.90484985763062e-11 650.75849014748 -860.682708058319;-0.00032 1.7854917086133e-11 663.662594444115 -850.772130439644;-0.00028 1.66572755417886e-11 676.415787589956 -840.668094575253;-0.00024 1.54558462766323e-11 689.01516961886 -830.372898035768;-0.0002 1.42509024853183e-11 701.457875540006 -819.888881860101;-0.00016 1.30427181616736e-11 713.74107598937 -809.21843002312;-0.00012 1.18315680363945e-11 725.861977873095 -798.363968893554;-8e-05 1.06177275145751e-11 737.817825002619 -787.327966682259;-4e-05 9.40147261308224e-12 749.605898721407 -776.112932880968]  x5=0.00139688767047948  V1=ones(3,3)  V2=ones(3,3)  I1=ones(3,3)  I2=ones(3,3)  nHarmo=1  Measurements=None
      settings: AttributesFormatString=\n  SourceProductName=Simscape Power Systems
  SAG7 : powerlib/Measurements/Three-Phase V-I Measurement  VoltageMeasurement=no  SetLabelV=on  LabelV=Vabc_SAG7  Vpu=on  VpuLL=off  CurrentMeasurement=no  SetLabelI=off  LabelI=Iabc_SAG7  Ipu=off  Pbase=100e6  Vbase=735e3  OutputType=Magnitude  PhasorSimulation=off  PSBequivalent=0
  Scope4 : Scope
  Scope5 : Scope
  Scope6 : Scope
  Subsystem : Subsystem
      mask Display: disp('Display\nWaveforms')
  Subsystem1 : Subsystem
      mask Display: disp('PSS_select')
  Subsystem2 : Subsystem
      settings: OpenFcn=LoadFlow_VSC
      mask Display: color('blue'),disp('Update Loadflow')
  VSC00 : Subsystem  mask(VSC){fb=fb, Sn=VSC01_Sn, Pn=VSC01_Pn, Un1=VSC01_Un1, Un2=VSC01_Un2, Rt_pu=VSC01_Rt_pu, Lt_pu=VSC01_Lt_pu, Rm_pu=500, Lm_pu=0, Lf_pu=VSC01_Lf_pu, Rf_pu=VSC01_Rf_pu, Cf_pu=VSC01_Cf_pu, Tr_PLL=VSC01_Tr_PLL, Val_Freq_Support=on, Val_gamma=on, R_percent=VSC01_R, Rv=VSC01_Rv, W_TVR=VSC01_W_LF, gainpopup=3, wc1=VSC01_wc1, mp1=VSC01_mp1, wc2=VSC01_wc2, mp2=VSC01_mp2, wc3=VSC01_wc3, mp3=VSC01_mp3, T1=VSC01_T1, T2=VSC01_T2, LFpopup=PV, P0=0.9, Q0=-0.23664, V0=1, Theta0=-20.9762, innercontrol=1, Ki_i=1.19, Kp_i=0.73, Kp_v=0.52, Ki_v=1.16, Kffv=1, Kffi=1, I_max=1.25}
      mask prompts: fb "Nominal Frequency (Hz)"; Sn "Nominal Apparent Power (VA)"; Pn "Nominal Power (W)"; Un1 "VSC side Nominal Ph-Ph Voltage (V)"; Un2 "Grid side Nominal Ph-Ph Voltage (V)"; Rt_pu "R (pu)"; Lt_pu "L (pu)"; Rm_pu "Rm (pu)"; Lm_pu "Lm (pu)"; Lf_pu "Lf (pu)"; Rf_pu "Rf (pu)"; Cf_pu "Cf (pu)"; Tr_PLL "Time response (s)"; Val_Freq_Support "Frequency Support"; Val_gamma "gamma activation"; R_percent "Droop Gain (%)"; Rv "Damping Resistance (Rv)"; W_TVR "Dr filter"; gainpopup "Strategy"; wc1 "wc"; mp1 "mp"; wc2 "wc"; mp2 "mp"; wc3 "wc"; mp3 "mp"; P0 "Initial Active Power (pu)"; Q0 "Initial Reactive Power (pu)"; V0 "Initial Voltage (pu)"; Theta0 "Initial Angle (°)"; innercontrol "Strategy"
      mask init:
      | % Update Name of LF bus for internal purpose
      |     NameStr = [get_param(gcb,'Name')];% '_LF'];
      |     set_param([gcb '/Load Flow Bus'],'ID',NameStr);
      |     %disp(NameStr);
      |     
      | % Increase size of Mask dialog box
      |    % pause(0.1);
      |     
      |     
      | % Base values
      |     %Un = Un1;
      |     Pb = Pn;
      |     cos_phi_n = Pn/Sn;
      |     Sb = Pb/cos_phi_n;
      |     %Ub = Un;
      |     Vn = Un1/sqrt(3);
      |     Vb = Vn;
      |     %Ib = Sb / Ub;
      |     Ib = Sb / (3*Vb);
      |     Zb = (3*Vb^2)/Sb;
      |     wb = 2*pi*fb;
      |     Lb = Zb/wb;
      |     Cb = 1/(Zb*wb);
      |   
      | % PLL derivation of the parameters
      |     wn_PLL=5/Tr_PLL;
      |     zeta_PLL = 1;
      |     Kp_PLL_pu = 2*zeta_PLL*wn_PLL/wb;
      |     Ki_PLL_pu = wn_PLL^2/wb;
      |     
      | % Set the chosen strategy
      |     Chosen_Strategy = gainpopup;
      |     
      | % Set the frequency droop gain
      |     R = R_percent;
      | 
      | % Compute Initial Voltage of VSC 
      | %   from steady-state output transformer model and Loadflow result
      |     if (LFpopup == 'PQ')
      |         V0 = 1;
      |     end
      |         
      |     R1_pu = Rt_pu/2;
      |     L1_pu = Lt_pu/2;
      |     R2_pu = Rt_pu/2;
      |     L2_pu = Lt_pu/2;
      |     X1_pu = L1_pu;
      |     X2_pu = L2_pu;
      |     Xm_pu = Lm_pu;
      |     
      |     Zm_pu = 1/(1/Rm_pu);
      | 
      |     S0=P0+1i*Q0;
      |     I2 = conj(S0)/(V0);
      | 
      |     Vm = (R2_pu+1i*X2_pu)*I2 + V0;
      |     Im = Vm/Zm_pu;
      | 
      |     I1 = I2 + Im;
      |     V1 = (R1_pu+1i*X1_pu) * I1 + Vm;
      | 
      |     Vvsc0 = abs(V1);
      |    % disp(Vvsc0*1000)
      |     Theta_vsc0 = angle(V1) * 180/pi+Theta0;
      |         
      |     %vd0=Vvsc0*cos(Theta0*2*pi/180);
      |     %vq0=Vvsc0*sin(Theta0*2*pi/180); 
      |  
      |     %Va0 = Vvsc0*sqrt(2)*Ub/sqrt(3)*sin(Theta_vsc0*pi/180);
      |     %Vb0 = Vvsc0*sqrt(2)*Ub/sqrt(3)*sin(Theta_vsc0*pi/180-2*pi/3);
      |     %Vc0 = Vvsc0*sqrt(2)*Ub/sqrt(3)*sin(Theta_vsc0*pi/180+2*pi/3);
      |     
      |     Va0 = Vvsc0*sqrt(2)*Vb*sin(Theta_vsc0*pi/180);
      |     Vb0 = Vvsc0*sqrt(2)*Vb*sin(Theta_vsc0*pi/180-2*pi/3);
      |     Vc0 = Vvsc0*sqrt(2)*Vb*sin(Theta_vsc0*pi/180+2*pi/3);
      |     
      | % Generate string to display LF results on Mask
      |     %str_tmp = fprintf("Vvsc0 = %d, Theta_vsc0 = %d°",Vvsc0,Theta_vsc0);
      |     mo = get_param(gcb,'MaskObject');
      |     mo.getDialogControl('LF_vsc_str').Prompt = ['V0 = ', num2str(Vvsc0),' pu, Angle = ', num2str(Theta_vsc0),'°'];
      |     mo.getDialogControl('LF_pcc_str').Prompt = ['V0 = ', num2str(V0),' pu, Angle = ', num2str(Theta0),'°'];
      |     mo.getDialogControl('LF_pcc_Power_str').Prompt = ['P0 = ', num2str(P0),' pu, Q0 = ', num2str(Q0),' pu'];
      |     %set_param([gcb],'LF_str',str_tmp);
      |  %GRD00_Theta0 = Theta0;
      |  %P0 = 200e6;
      |  %Q0 = 0;
      |  % Initial current values of VSC (dq pu) 
      |  %id0 =(P0*vd0+Q0*vq0)/(vd0^2+vq0^2) * 1/Ib; %
      |  %iq0 =(P0*vq0-Q0*vd0)/(vd0^2+vq0^2) * 1/Ib; %Initial current in the connexion inductance
      settings: OpenFcn=|
      | NameStr = get_param(gcb,'Name');
      | open_system(gcbh, 'Mask');
      | 
      | h2AllOpenDlgs = DAStudio.ToolRoot.getOpenDialogs;
      | 
      | for i=1:length(h2AllOpenDlgs)
      |     try
      |          %disp(h2AllOpenDlgs(i).getSource.getBlock.Name);
      |         Dialog_block_name = h2AllOpenDlgs(i).getSource.getBlock.Name;
      |          %strcmp(Dialog_block_name, NameStr),
      |         if (strcmp(h2AllOpenDlgs(i).getSource.getBlock.Name, NameStr))
      |             iPos = h2AllOpenDlgs(i).position;
      |             h2AllOpenDlgs(i).position = [iPos(1)   iPos(2)   iPos(3)*1.6   iPos(4)];
      |         end
      |     end
      | end
      mask TypeOptions gainpopup: 1 | 2 | 3
      mask Callback gainpopup:
      | % Get the mask parameter values. This is a cell
      | %   array of character vectors.
      | maskStr = get_param(gcb,'gainpopup');
      | p=Simulink.Mask.get(gcb);
      | 
      | % The pop-up menu is the first mask parameter.
      | %   Check the value selected in the pop-up
      | if strcmp(maskStr,'1'),
      | 
      |     % Set the visibility of both parameters on when
      |     %   User-defined is selected in the pop-up.
      |     p.getDialogControl('Param_Strat_1').Visible='on';
      |     p.getDialogControl('Param_Strat_2').Visible='off';
      |     p.getDialogControl('Param_Strat_3').Visible='off';
      | 
      | 
      | elseif strcmp(maskStr,'2'),
      | 
      |     % Set the visibility of both parameters on when
      |     %   User-defined is selected in the pop-up.
      |     p.getDialogControl('Param_Strat_1').Visible='off';
      |     p.getDialogControl('Param_Strat_2').Visible='on';
      |     p.getDialogControl('Param_Strat_3').Visible='off';
      | 
      | 
      |     % Turn off the visibility of the Value field
      |     %   when User-defined is not selected.
      | elseif strcmp(maskStr,'3'),
      | 
      |     % Set the visibility of both parameters on when
      |     %   User-defined is selected in the pop-up.
      |     p.getDialogControl('Param_Strat_1').Visible='off';
      |     p.getDialogControl('Param_Strat_2').Visible='off';
      |     p.getDialogControl('Param_Strat_3').Visible='on';
      | 
      | else
      | 
      |     % Set the visibility of both parameters on when
      |     %   User-defined is selected in the pop-up.
      |     p.getDialogControl('Param_Strat_1').Visible='off';
      |     p.getDialogControl('Param_Strat_2').Visible='off';
      |     p.getDialogControl('Param_Strat_3').Visible='off';
      | 
      | end
      mask TypeOptions LFpopup: Swing | PQ | PV
      mask Callback LFpopup:
      | % Get the mask parameter values. This is a cell
      | %   array of character vectors.
      | maskStr = get_param(gcb,'LFpopup');
      | p=Simulink.Mask.get(gcb);
      | 
      | % The pop-up menu is the first mask parameter.
      | %   Check the value selected in the pop-up
      | if strcmp(maskStr,'Swing'),
      | 
      |     % Set the visibility of both parameters on when
      |     %   User-defined is selected in the pop-up.
      |     p.getParameter('P0').Visible='off';
      |     p.getParameter('Q0').Visible='off';
      |     p.getParameter('V0').Visible='on';
      |     p.getParameter('Theta0').Visible='on';
      |     set_param([gcb '/Source_For_LF'],'BusType','swing');
      | 
      | elseif strcmp(maskStr,'PQ'),
      | 
      |     % Set the visibility of both parameters on when
      |     %   User-defined is selected in the pop-up.
      |     p.getParameter('P0').Visible='on';
      |     p.getParameter('Q0').Visible='on';
      |     p.getParameter('V0').Value='1';
      |     set_param(gcb,'V0','1');
      |     p.getParameter('V0').Visible='off';
      |     p.getParameter('Theta0').Visible='off';
      |     set_param([gcb '/Source_For_LF'],'BusType','PQ');
      | 
      |     % Turn off the visibility of the Value field
      |     %   when User-defined is not selected.
      | else
      | 
      |     % Set the visibility of both parameters on when
      |     %   User-defined is selected in the pop-up.
      |     p.getParameter('P0').Visible='on';
      |     p.getParameter('Q0').Visible='off';
      |     p.getParameter('V0').Visible='on';
      |     p.getParameter('Theta0').Visible='off';
      |     set_param([gcb '/Source_For_LF'],'BusType','PV');
      | 
      | end
      mask TypeOptions innercontrol: 1
      mask Callback innercontrol:
      | % Get the mask parameter values. This is a cell
      | %   array of character vectors.
      | maskStr = get_param(gcb,'innercontrol');
      | p=Simulink.Mask.get(gcb);
      | 
      | % The pop-up menu is the first mask parameter.
      | %   Check the value selected in the pop-up
      | if strcmp(maskStr,'1'),
      | 
      |     % Set the visibility of both parameters on when
      |     %   User-defined is selected in the pop-up.
      |     p.getDialogControl('Param_Strat_11').Visible='on';
      | 
      | 
      | else
      | 
      |     % Set the visibility of both parameters on when
      |     %   User-defined is selected in the pop-up.
      |     p.getDialogControl('Param_Strat_11').Visible='on';
      | 
      | end
      mask DialogControl Nominal_Param Prompt: Nominal Value
      mask DialogControl Container20 Prompt: Output Transformer and filter
      mask DialogControl Container31 Prompt: Transformer
      mask DialogControl Container32 Prompt: Filter
      mask DialogControl Control_Param Prompt: Control Parameter
      mask DialogControl Container13 Prompt: PLL
      mask DialogControl Container14 Prompt: Frequency Support
      mask DialogControl Container15 Prompt: Transient Virtual Resistor
      mask DialogControl Container18 Prompt: Control Strategy
      mask DialogControl Title_Strat_1 Prompt: Strategy 1
      mask DialogControl Title_Strat_2 Prompt: Strategy 2
      mask DialogControl Title_Strat_3 Prompt: Strategy 3
      mask DialogControl LF_Param Prompt: Loadflow
      mask DialogControl Control4 Prompt: Initial Operating Point
      mask DialogControl Container24 Prompt: VSC side
      mask DialogControl LF_vsc_str Prompt: V0 = 0.97854 pu, Angle = -12.9677°
      mask DialogControl Container25 Prompt: PCC
      mask DialogControl LF_pcc_str Prompt: V0 = 1 pu, Angle = -20.9762°
      mask DialogControl LF_pcc_Power_str Prompt: P0 = 0.9 pu, Q0 = -0.23664 pu
      mask DialogControl UpdateLoadflow Prompt: Update Loadflow
      mask DialogControl UpdateLoadflow Callback: Load_Flow_VSC
      mask DialogControl Container21 Prompt: Inner control
      mask DialogControl Title_Strat_11 Prompt: Cascaded_control
  dE_set : Constant  Value=0
  powergui : powerlib/powergui  Priority=1  SimulationMode=Discrete  SampleTime=Time_Step  frequency=60  Iterations=50  frequencyindice=60  Pbase=1e+008  ErrMax=0.0001  UnitsV=kV  UnitsW=MW  buscounter=0  FunctionMessages=off  echomessages=off  EnableUseOfTLC=off  CurrentSourceSwitches=off  DisableSnubberDevices=off  DisableRonSwitches=off  DisableVfSwitches=off  DisplayEquations=off  SolverType=Tustin/Backward Euler (TBE)  Interpol=off  ExternalGateDelay=off  methode=off  Ts=100  x0status=blocks  SPID=off  SwTol=0  HookPort=off  RestoreLinks=warning  ResistiveCurrentMeasurement=off  Frange=[0:2:500]  Ylog=off  Xlog=on  ShowGrid=off  save=off  variable=ZData  structure=0  ZoomFFT=off  StartTime=0.0  cycles=1  DisplayStyle=1  fundamental=60  FreqAxis=off  MaxFrequency=1000  frequencyindicesteady=1  RmsSteady=1  display=off
  wires:
  PSS/1 -> Subsystem1/1(In1)
  D_Pset/1 -> VSC00/2(dP_set (pu))
  dE_set/1 -> VSC00/1(dE_set (pu))
  Bus Selector1/3 -> Scope6/1  "<f>"
  Bus Selector1/2 -> Scope5/1  "<Q>"
  VSC00/1(m) -> Bus Selector1/1
  Bus Selector1/1 -> Scope4/1  "<P>"
  connections:
  QUE Load and Wind Generation/LConn3 -- MTL-QUE 5*219km/RConn3 -- Load Flow Bus2/LConn1 -- CHM-JCA 2*252km/RConn3 -- QUE7/LConn3
  MTL7/RConn1 -- MTL-QUE 5*219km/LConn1
  MTL7/RConn2 -- MTL-QUE 5*219km/LConn2
  MTL7/RConn3 -- MTL-QUE 5*219km/LConn3
  QUE Load and Wind Generation/LConn2 -- MTL-QUE 5*219km/RConn2 -- CHM-JCA 2*252km/RConn2 -- QUE7/LConn2
  QUE Load and Wind Generation/LConn1 -- MTL-QUE 5*219km/RConn1 -- CHM-JCA 2*252km/RConn1 -- QUE7/LConn1
  Cs SAG/LConn1 -- SAG7/RConn1 -- SAG 660Mvar/LConn1
  Cs SAG/LConn2 -- SAG7/RConn2 -- SAG 660Mvar/LConn2
  Cs SAG/LConn3 -- SAG7/RConn3 -- SAG 660Mvar/LConn3
  Load Flow Bus3/LConn1 -- CHM-SAG 117km/RConn3 -- SAG7/LConn3
  Cs CHMS/LConn1 -- CHM-SAG 117km/LConn1 -- North-West Network/RConn4
  Cs CHMS/LConn2 -- CHM-SAG 117km/LConn2 -- North-West Network/RConn5
  Cs CHMS/LConn3 -- CHM-SAG 117km/LConn3 -- North-West Network/RConn6
  Cs SAG/RConn1 -- SAG-MIC 247km/LConn1
  Cs SAG/RConn3 -- SAG-MIC 247km/LConn3
  Cs CHMS/RConn3 -- CHM-JCA 2*252km/LConn3
  Cs CHMS/RConn2 -- CHM-JCA 2*252km/LConn2
  Cs CHMS/RConn1 -- CHM-JCA 2*252km/LConn1
  Cs SAG/RConn2 -- SAG-MIC 247km/LConn2
  SAG7/LConn2 -- CHM-SAG 117km/RConn2
  SAG7/LConn1 -- CHM-SAG 117km/RConn1
  SAG-MIC 247km/RConn1 -- North_East Network/LConn1
  SAG-MIC 247km/RConn2 -- North_East Network/LConn2
  SAG-MIC 247km/RConn3 -- North_East Network/LConn3
  QUE7/RConn1 -- North_East Network/LConn4
  QUE7/RConn2 -- North_East Network/LConn5
  QUE7/RConn3 -- North_East Network/LConn6
  MTL7/LConn1 -- MTL Load/LConn1 -- VSC00/RConn1 -- North-West Network/RConn1
  MTL7/LConn2 -- MTL Load/LConn2 -- VSC00/RConn2 -- North-West Network/RConn2
  MTL7/LConn3 -- MTL Load/LConn3 -- VSC00/RConn3 -- North-West Network/RConn3
